simulink model "SimulinkschaltbildTeil3MatlabFunctions"  (R2014b)
settings: Solver=ode3  StartTime=0.0  StopTime=120.0  FixedStep=0.002  RelTol=1e-3
settings Model: Creator=Florian  LastModifiedBy=Florian

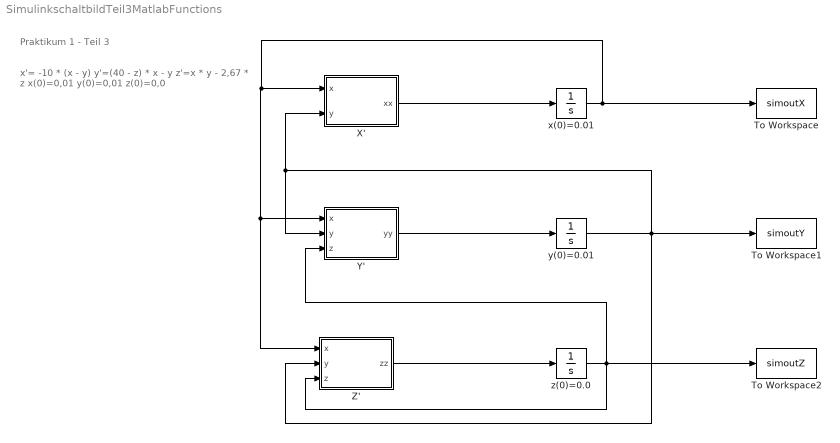
== system SimulinkschaltbildTeil3MatlabFunctions ==
  note: Praktikum 1 - Teil 3
  note: x'= -10 * (x - y)
      | y'=(40 - z) * x - y
      | z'=x * y - 2,67 * z
      |
      | x(0)=0,01 y(0)=0,01 z(0)=0,0
  To Workspace : ToWorkspace  VariableName=simoutX  SampleTime=-1
  To Workspace1 : ToWorkspace  VariableName=simoutY  SampleTime=-1
  To Workspace2 : ToWorkspace  VariableName=simoutZ  SampleTime=-1
  X' : MATLAB Function  TreatAsAtomicUnit=on
  Y' : MATLAB Function  TreatAsAtomicUnit=on
  Z' : MATLAB Function  TreatAsAtomicUnit=on
  x(0)=0.01 : Integrator  InitialCondition=0.01
  y(0)=0.01 : Integrator  InitialCondition=0.01
  z(0)=0.0 : Integrator
  wires:
  X'/1(xx) -> x(0)=0.01/1
  x(0)=0.01/1 -> To Workspace/1, Z'/1(x), Y'/1(x), X'/1(x)
  y(0)=0.01/1 -> X'/2(y), Y'/2(y), To Workspace1/1, Z'/2(y)
  Y'/1(yy) -> y(0)=0.01/1
  z(0)=0.0/1 -> Y'/3(z), To Workspace2/1, Z'/3(z)
  Z'/1(zz) -> z(0)=0.0/1

== matlab function SimulinkschaltbildTeil3MatlabFunctions/Y' ==
  data: x input; y input; z input; yy output
function yy = fcn(x,y,z)
yy=(40-z)*x-y;

== matlab function SimulinkschaltbildTeil3MatlabFunctions/X' ==
  data: x input; y input; xx output
function xx = fcn(x,y)
xx=-10*(x-y);

== matlab function SimulinkschaltbildTeil3MatlabFunctions/Z' ==
  data: x input; y input; z input; zz output
function zz = fcn(x,y,z)
zz=x*y-2.67*z;
